simulink model "HMI_V2"  (R2023a)
settings: Solver=VariableStepAuto  StartTime=0.0  StopTime=10.0  RelTol=1e-3
undefined symbols (not defined in the file or in its folder): An, ETATH, Fn, P0, P1, P2, P21, P3, P31, P4, P41, P415, P5, Ps, Q, rho, SFC, T0, T1, T2, T21, T3, T31, T41, T415, T5, Ts, Vj, W1, W2, W21, W3, W31, W4, W41, W415, W5, WHPC, WLPC
settings Model: Creator=martn  LastModifiedBy=martn

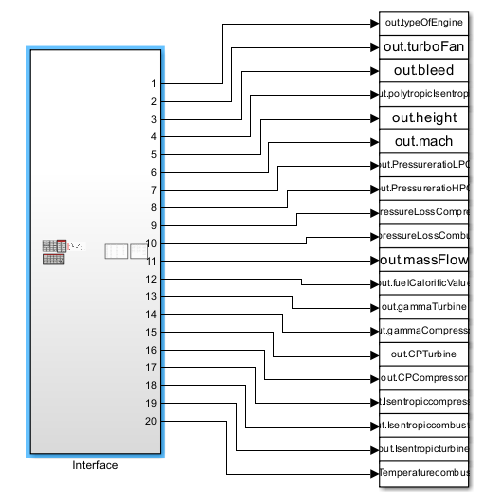
[thumbnail: Simulink's stored preview of the top-level diagram]
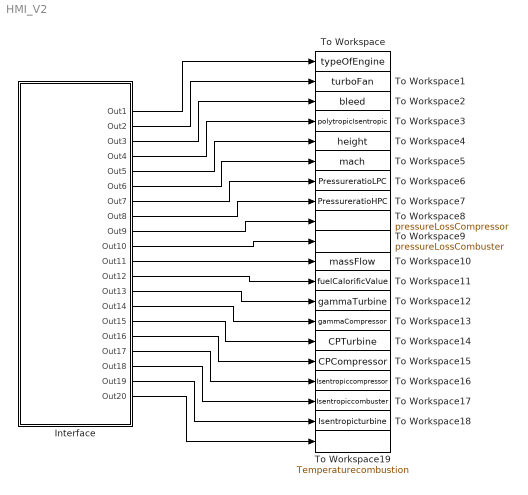
== system HMI_V2 ==
  Interface : Subsystem
  To Workspace : ToWorkspace  VariableName=typeOfEngine  SampleTime=-1
  To Workspace1 : ToWorkspace  VariableName=turboFan  SampleTime=-1
  To Workspace10 : ToWorkspace  VariableName=massFlow  SampleTime=-1
  To Workspace11 : ToWorkspace  VariableName=fuelCalorificValue  SampleTime=-1
  To Workspace12 : ToWorkspace  VariableName=gammaTurbine  SampleTime=-1
  To Workspace13 : ToWorkspace  VariableName=gammaCompressor  SampleTime=-1
  To Workspace14 : ToWorkspace  VariableName=CPTurbine  SampleTime=-1
  To Workspace15 : ToWorkspace  VariableName=CPCompressor  SampleTime=-1
  To Workspace16 : ToWorkspace  VariableName=Isentropiccompressor  SampleTime=-1
  To Workspace17 : ToWorkspace  VariableName=Isentropiccombuster  SampleTime=-1
  To Workspace18 : ToWorkspace  VariableName=Isentropicturbine  SampleTime=-1
  To Workspace19 : ToWorkspace  VariableName=Temperaturecombustion  SampleTime=-1
  To Workspace2 : ToWorkspace  VariableName=bleed  SampleTime=-1
  To Workspace3 : ToWorkspace  VariableName=polytropicIsentropic  SampleTime=-1
  To Workspace4 : ToWorkspace  VariableName=height  SampleTime=-1
  To Workspace5 : ToWorkspace  VariableName=mach  SampleTime=-1
  To Workspace6 : ToWorkspace  VariableName=PressureratioLPC  SampleTime=-1
  To Workspace7 : ToWorkspace  VariableName=PressureratioHPC  SampleTime=-1
  To Workspace8 : ToWorkspace  VariableName=pressureLossCompressor  SampleTime=-1
  To Workspace9 : ToWorkspace  VariableName=pressureLossCombuster  SampleTime=-1
  wires:
  Interface/1(Out1) -> To Workspace/1
  Interface/2(Out2) -> To Workspace1/1
  Interface/3(Out3) -> To Workspace2/1
  Interface/4(Out4) -> To Workspace3/1
  Interface/5(Out5) -> To Workspace4/1
  Interface/6(Out6) -> To Workspace5/1
  Interface/7(Out7) -> To Workspace6/1
  Interface/8(Out8) -> To Workspace7/1
  Interface/9(Out9) -> To Workspace8/1
  Interface/10(Out10) -> To Workspace9/1
  Interface/11(Out11) -> To Workspace10/1
  Interface/12(Out12) -> To Workspace11/1
  Interface/13(Out13) -> To Workspace12/1
  Interface/14(Out14) -> To Workspace13/1
  Interface/15(Out15) -> To Workspace14/1
  Interface/16(Out16) -> To Workspace15/1
  Interface/17(Out17) -> To Workspace16/1
  Interface/18(Out18) -> To Workspace17/1
  Interface/19(Out19) -> To Workspace18/1
  Interface/20(Out20) -> To Workspace19/1

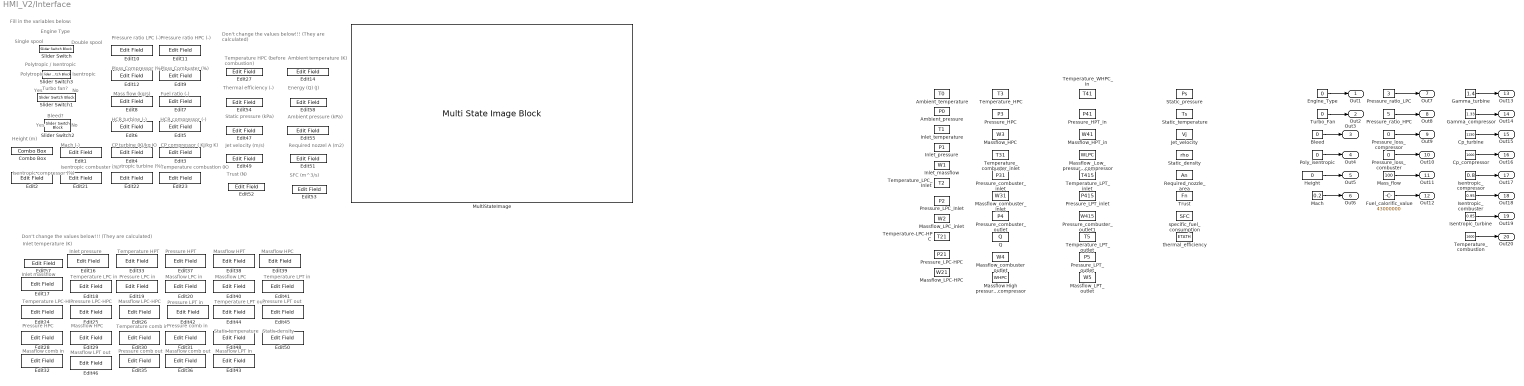
== system HMI_V2/Interface ==
  note: Don't change the values below!!! (They are calculated)
  note: Single spool
  note: Engine Type
  note: Double spool
  note: Turbo fan?
  note: Yes
  note: No
  note: Bleed?
  note: No
  note: Yes
  note: Polytropic / Isentropic
  note: Polytropic
  note: Isentropic
  note: Pressure ratio LPC
      | (-)
  note: Fill in the variables below:
  note: Inlet pressure
  note: Inlet massflow
  note: Temperature LPC in
  note: Pressure LPC in
  note: Massflow LPC in
  note: Temperature LPC-HPC
  note: Pressure LPC-HPC
  note: Massflow LPC-HPC
  note: Pressure HPC
  note: Massflow HPC
  note: Temperature comb in
  note: Pressure comb in
  note: Massflow comb in
  note: Pressure comb out
  note: Massflow comb out
  note: Temperature HPT
  note: Pressure HPT
  note: Massflow HPT
  note: Massflow HPC
  note: Massflow LPC
  note: Temperature LPT in
  note: Pressure LPT in
  note: Massflow LPT in
  note: Temperature LPT out
  note: Pressure LPT out
  note: Massflow LPT out
  note: Static temperature
  note: Static density
  note: Pressure ratio HPC
      | (-)
  note: Ploss Compressor
      | (%)
  note: Ploss Combuster
      | (%)
  note: Mass flow
      | (kg/s)
  note: Fuel ratio
      | (-)
  note: HCR turbine
      | (-)
  note: HCR compressor
      | (-)
  note: CP turbine
      | (KJ/kg K)
  note: CP compressor
      | ( KJ/kg K)
  note: Isentropic turbine
      | (%)
  note: Temperature combustion (K)
  note: Isentropic combuster (%)
  note: Isentropic compressor (%)
  note: Mach
      | (-)
  note: Height
      | (m)
  note: Ambient pressure
      | (kPa)
  note: Ambient temperature
      | (K)
  note: Inlet temperature
      | (K)
  note: Don't change the values below!!! (They are calculated)
  note: Temperature HPC (before combustion)
  note: Energy (Q)
      | (J)
  note: Static pressure
      | (kPa)
  note: Required nozzel A
      | (m2)
  note: Jet velocity
      | (m/s)
  note: Trust
      | (N)
  note: SFC
      | (m^3/s)
  note: Thermal efficiency
      | (-)
  Ambient_pressure : Constant  Value=P0
  Ambient_temperature : Constant  Value=T0
  Bleed : Constant  Value=0
  Combo Box : ComboBox  LabelPosition=Hide  SelectedLabel=0m
      settings: Values={{'0m', '250m', '500m', '750m', '1000m', '1250m', '1500m', '1750m', '2000m', '2250m', '2500m', '2750m', '3000m', '3250m', '3500m', '3750m', '4000m', '4250m', '4500m', '4750m', '5000m', '5250m', '5500m', '5750m', '6000m'}, [0 250 500 750 1000 1250 1500 1750 2000 2250 2500 2750 3000 3250 3500 3750 4000 4250 4500 4750 5000 5250 5500 5750 6000]}
  Cp_compressor : Constant  Value=1000
  Cp_turbine : Constant  Value=1150
  Edit{1..12,14,16..33,35..55,57..58} (54 alike) : EditField  LabelPosition=Hide  ShowInitialText=on  Alignment=Center
  Engine_Type : Constant  Value=0
  Fuel_calorific_value : Constant  Value=43000000
  Gamma_compressor : Constant  Value=1.33
  Gamma_turbine : Constant  Value=1.4
  Height : Constant  Value=0
  Inlet_massflow : Constant  Value=W1
  Inlet_pressure : Constant  Value=P1
  Inlet_temperature : Constant  Value=T1
  Isentropic_combuster : Constant  Value=0.95
  Isentropic_compressor : Constant  Value=0.8
  Isentropic_turbine : Constant  Value=0.85
  Jet_velocity : Constant  Value=Vj
  Mach : Constant  Value=0.2
  Mass_flow : Constant  Value=100
  Massflow High pressure compressor : Constant  Value=WHPC
  Massflow _Low_pressure_compressor : Constant  Value=WLPC
  Massflow_HPC : Constant  Value=W3
  Massflow_HPT_in : Constant  Value=W41
  Massflow_LPC-HPC : Constant  Value=W21
  Massflow_LPC_inlet : Constant  Value=W2
  Massflow_LPT_outlet : Constant  Value=W5
  Massflow_combuster outlet : Constant  Value=W4
  Massflow_combuster_inlet : Constant  Value=W31
  MultiStateImage : MultiStateImageBlock  LabelPosition=Hide
  Poly_isentropic : Constant  Value=0
  Pressure_HPC : Constant  Value=P3
  Pressure_HPT_in : Constant  Value=P41
  Pressure_LPC-HPC : Constant  Value=P21
  Pressure_LPC_Inlet : Constant  Value=P2
  Pressure_LPT_inlet : Constant  Value=P415
  Pressure_LPT_outlet : Constant  Value=P5
  Pressure_combuster_inlet : Constant  Value=P31
  Pressure_combuster_outlet : Constant  Value=P4
  Pressure_combuster_outlet1 : Constant  Value=W415
  Pressure_loss_combuster : Constant  Value=0
  Pressure_loss_compressor : Constant  Value=0
  Pressure_ratio_HPC : Constant  Value=5
  Pressure_ratio_LPC : Constant  Value=3
  Q : Constant  Value=Q
  Required_nozzle_area : Constant  Value=An
  Slider Switch{,1..3} (4 alike) : SliderSwitchBlock  LabelPosition=Hide
      settings: Values={{'', ''}, [0 1]}
  Static_density : Constant  Value=rho
  Static_pressure : Constant  Value=Ps
  Static_temperature : Constant  Value=Ts
  Temperature-LPC-HPC : Constant  Value=T21
  Temperature_HPC : Constant  Value=T3
  Temperature_LPC_Inlet : Constant  Value=T2
  Temperature_LPT_inlet : Constant  Value=T415
  Temperature_LPT_outlet : Constant  Value=T5
  Temperature_WHPC_In : Constant  Value=T41
  Temperature_combuster_inlet : Constant  Value=T31
  Temperature_combustion : Constant  Value=1600
  Trust : Constant  Value=Fn
  Turbo_Fan : Constant  Value=0
  specific_fuel_consumption : Constant  Value=SFC
  thermal_efficiency : Constant  Value=ETATH
  Out1 : Outport
  Out2 : Outport  Port=2
  Out3 : Outport  Port=3
  Out4 : Outport  Port=4
  Out5 : Outport  Port=5
  Out6 : Outport  Port=6
  Out7 : Outport  Port=7
  Out8 : Outport  Port=8
  Out9 : Outport  Port=9
  Out10 : Outport  Port=10
  Out11 : Outport  Port=11
  Out12 : Outport  Port=12
  Out13 : Outport  Port=13
  Out14 : Outport  Port=14
  Out15 : Outport  Port=15
  Out16 : Outport  Port=16
  Out17 : Outport  Port=17
  Out18 : Outport  Port=18
  Out19 : Outport  Port=19
  Out20 : Outport  Port=20
  wires:
  Engine_Type/1 -> Out1/1
  Turbo_Fan/1 -> Out2/1
  Bleed/1 -> Out3/1
  Poly_isentropic/1 -> Out4/1
  Mach/1 -> Out6/1
  Pressure_ratio_LPC/1 -> Out7/1
  Pressure_ratio_HPC/1 -> Out8/1
  Pressure_loss_compressor/1 -> Out9/1
  Pressure_loss_combuster/1 -> Out10/1
  Mass_flow/1 -> Out11/1
  Fuel_calorific_value/1 -> Out12/1
  Cp_compressor/1 -> Out16/1
  Cp_turbine/1 -> Out15/1
  Gamma_compressor/1 -> Out14/1
  Gamma_turbine/1 -> Out13/1
  Height/1 -> Out5/1
  Isentropic_compressor/1 -> Out17/1
  Isentropic_combuster/1 -> Out18/1
  Isentropic_turbine/1 -> Out19/1
  Temperature_combustion/1 -> Out20/1
